simulink model "model51"  (R2024a)
settings: Solver=VariableStepAuto  StartTime=0.0  StopTime=80  MaxStep=0.01  RelTol=1e-3
values from neighbouring files (symbols this model uses):
  ki = k_combinations(i, 1)    [script51.m]    (also in script52.m)
  kp = k_combinations(i, 2)    [script51.m]    (also in script52.m)
settings Model: Creator=eva  LastModifiedBy=eva

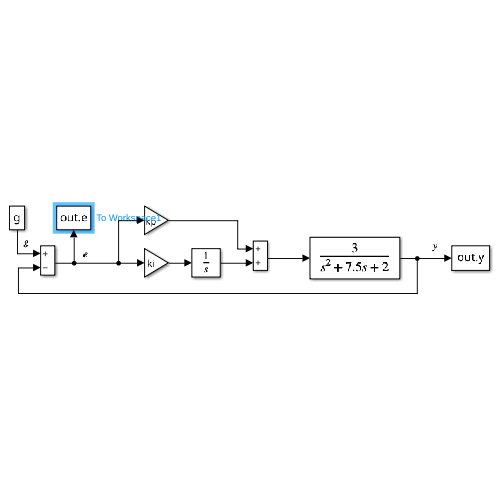
[thumbnail: Simulink's stored preview of the top-level diagram]
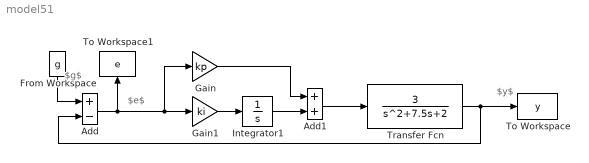
== system model51 ==
  note: $y$
  note: $g$
  note: $e$
  Add : Sum  Inputs=+-
  Add1 : Sum
  From Workspace : FromWorkspace  VariableName=g
  Gain : Gain  Gain=kp
  Gain1 : Gain  Gain=ki
  Integrator1 : Integrator
  To Workspace : ToWorkspace  VariableName=y  SaveFormat=Structure With Time  SampleTime=-1
  To Workspace1 : ToWorkspace  VariableName=e  SaveFormat=Structure With Time  SampleTime=-1
  Transfer Fcn : TransferFcn  Numerator=[3]  Denominator=[1 7.5 2]
  wires:
  From Workspace/1 -> Add/1
  Transfer Fcn/1 -> Add/2, To Workspace/1
  Add/1 -> Gain1/1, Gain/1, To Workspace1/1
  Add1/1 -> Transfer Fcn/1
  Gain1/1 -> Integrator1/1
  Integrator1/1 -> Add1/2
  Gain/1 -> Add1/1
